simulink model "quantizer_non_uniform"  (Simulink 8.7)
settings: Solver=FixedStepDiscrete  SolverMode=SingleTasking  StartTime=0.0  StopTime=1  FixedStep=1/10000  RelTol=1e-3  AbsTol=1e-6
values from neighbouring files (symbols this model uses):
  k = 1/4.902/(sqrt(10^(atenuation_dB/10)))    [quant_non_uniform.m]    (also in quant_uniform.m; speech_quant_non_uniform.m = sqrt(10^(atenuation_dB/10)); speech_quant_uniform.m = sqrt(10^(atenuation_dB/10)))
libraries: commsrccod2 x2, dspquant2 x1
settings Model: Creator=amoura  LastModifiedBy=Artur Moura
settings DataIOCC: LimitDataPoints=off  SignalLoggingSaveFormat=ModelDataLogs
settings OptimizationCC: BlockReduction=off  BooleanDataType=off  ExpressionDepthLimit=2147483647  InitFltsAndDblsToZero=on
settings DebuggingCC: SaveWithParameterizedLinksMsg=none  SignalResolutionControl=TryResolveAllWithWarning  MultiTaskDSMMsg=warning  MultiTaskCondExecSysMsg=none  FcnCallInpInsideContextMsg=UseLocalSettings  StateNameClashWarn=warning
settings HardwareCC: TargetUnknown=on
settings RTWCC: TemplateMakefile=grt_unix.tmf
settings GRTTargetCC: TargetFcnLib=ansi_tfl_tmw.mat  ModelReferenceCompliant=off  CombineOutputUpdateFcns=off  MatFileLogging=off  GRTInterface=on

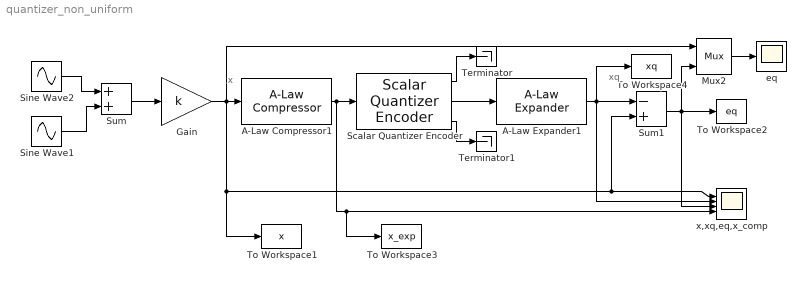
== system quantizer_non_uniform ==
  note: xq
  note: x
  A-Law Compressor1 : commsrccod2/A-Law Compressor  A=87.6  V=1
  A-Law Expander1 : commsrccod2/A-Law Expander  A=87.6  V=1
  Gain : Gain  Gain=k  SaturateOnIntegerOverflow=on  OutDataTypeStr=Inherit: Same as input  ParamDataTypeStr=Inherit: Same as input
  Mux2 : Mux  Inputs=2
  Scalar Quantizer Encoder : dspquant2/Scalar Quantizer Encoder  paramSrc=Specify via dialog  partType=Bounded  BBoundary=boundary  UBoundary=[2:9]  SearchMethod=Linear  tieBreakRule=Choose the lower index  outQU=on  outQError=on  codebook=codebook  outStatus=off  invalidin=Clip  idtype=int32  roundingMode=Floor  overflowMode=off
  Sine Wave1 : Sin  Amplitude=2  Frequency=2*pi*120  SampleTime=0
  Sine Wave2 : Sin  Amplitude=3  Frequency=2*pi*20  SampleTime=0
  Sum : Sum  SaturateOnIntegerOverflow=on  InputSameDT=on  OutDataTypeStr=Inherit: Same as first input
  Sum1 : Sum  Inputs=-+  SaturateOnIntegerOverflow=on  InputSameDT=on  OutDataTypeStr=Inherit: Same as first input
  Terminator : Terminator
  Terminator1 : Terminator
  To Workspace1 : ToWorkspace  VariableName=x  SampleTime=-1
  To Workspace2 : ToWorkspace  VariableName=eq  SampleTime=-1
  To Workspace3 : ToWorkspace  VariableName=x_exp  SampleTime=-1
  To Workspace4 : ToWorkspace  VariableName=xq  SampleTime=-1
  eq : Scope
  x,xq,eq,x_comp : Scope  NumInputPorts=4
  wires:
  Sum1/1 -> To Workspace2/1, Mux2/2, x,xq,eq,x_comp/3
  Gain/1 -> A-Law Compressor1/1, Mux2/1, x,xq,eq,x_comp/1, Sum1/2, To Workspace1/1
  Scalar Quantizer Encoder/2 -> A-Law Expander1/1
  Scalar Quantizer Encoder/3 -> Terminator1/1
  Scalar Quantizer Encoder/1 -> Terminator/1
  Sum/1 -> Gain/1
  Sine Wave1/1 -> Sum/2
  Sine Wave2/1 -> Sum/1
  A-Law Compressor1/1 -> Scalar Quantizer Encoder/1, To Workspace3/1, x,xq,eq,x_comp/4
  A-Law Expander1/1 -> To Workspace4/1, Sum1/1, x,xq,eq,x_comp/2
  Mux2/1 -> eq/1
